simulink model "modeloNaoLinear"  (R2022a)
settings: Solver=FixedStepAuto  StartTime=0.0  StopTime=15  FixedStep=0.01  RelTol=1e-3
values from neighbouring files (symbols this model uses):
  CA = 8.564    [Identificacao.m]    (also in Linearizacao_CSTR.m)
  CAf = 10    [Identificacao.m]    (also in Linearizacao_CSTR.m)
  dCAf = 0    [Identificacao.m]    (also in Linearizacao_CSTR.m)
  dF = 0.01    [Identificacao.m]    (also in Linearizacao_CSTR.m)
  dTf = 0    [Identificacao.m]    (also in Linearizacao_CSTR.m)
  dTj = 0    [Identificacao.m]    (also in Linearizacao_CSTR.m)
  F = 1    [Identificacao.m]    (also in Linearizacao_CSTR.m)
  T = 311.2    [Identificacao.m]    (also in Linearizacao_CSTR.m; modeloDegrau.m = -Theta(3); parametrosFOPTD_igor.m = -Theta(3))
  Tf = 298    [Identificacao.m]    (also in Linearizacao_CSTR.m)
  Tj = 298    [Identificacao.m]    (also in Linearizacao_CSTR.m)
settings Model: Creator=veloc  LastModifiedBy=veloc

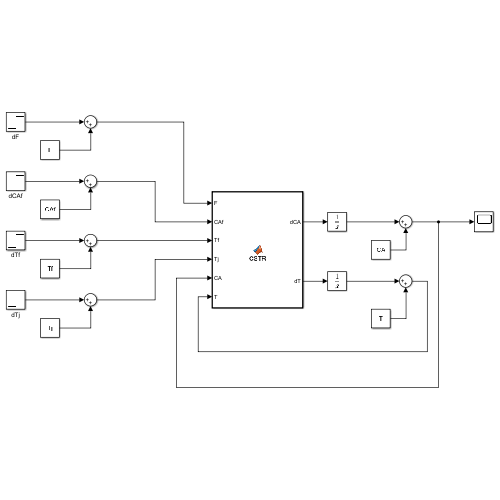
[thumbnail: Simulink's stored preview of the top-level diagram]
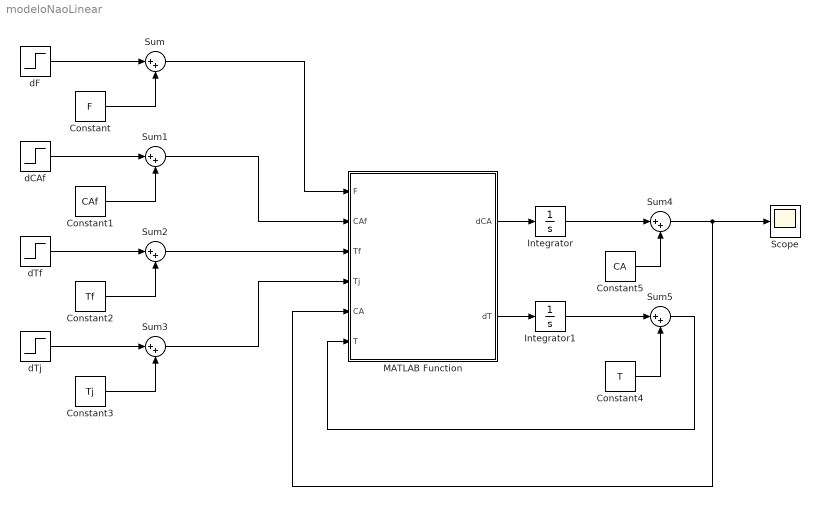
== system modeloNaoLinear ==
  Constant : Constant  Value=F
  Constant1 : Constant  Value=CAf
  Constant2 : Constant  Value=Tf
  Constant3 : Constant  Value=Tj
  Constant4 : Constant  Value=T
  Constant5 : Constant  Value=CA
  Integrator : Integrator
  Integrator1 : Integrator
  MATLAB Function : MATLAB Function  TreatAsAtomicUnit=on
  Scope : Scope
  Sum{,1..5} (6 alike) : Sum  Inputs=|++
  dCAf : Step  Time=0  Before=dCAf  SampleTime=0
  dF : Step  Time=0  After=dF  SampleTime=0
  dTf : Step  Time=0  After=dTf  SampleTime=0
  dTj : Step  Time=0  After=dTj  SampleTime=0
  wires:
  Sum3/1 -> MATLAB Function/4(Tj)
  Sum2/1 -> MATLAB Function/3(Tf)
  Sum1/1 -> MATLAB Function/2(CAf)
  Sum/1 -> MATLAB Function/1(F)
  Constant1/1 -> Sum1/2
  Constant/1 -> Sum/2
  Constant2/1 -> Sum2/2
  Constant3/1 -> Sum3/2
  Sum5/1 -> MATLAB Function/6(T)
  Constant4/1 -> Sum5/2
  Constant5/1 -> Sum4/2
  dF/1 -> Sum/1
  dCAf/1 -> Sum1/1
  dTf/1 -> Sum2/1
  dTj/1 -> Sum3/1
  Sum4/1 -> Scope/1, MATLAB Function/5(CA)
  MATLAB Function/2(dT) -> Integrator1/1
  MATLAB Function/1(dCA) -> Integrator/1
  Integrator/1 -> Sum4/1
  Integrator1/1 -> Sum5/1

== matlab function modeloNaoLinear/MATLAB Function ==
  data: F input; dCA output; CAf input; Tf input; Tj input; CA input; T input; dT output
function [dCA,dT] = CSTR(F, CAf, Tf, Tj, CA, T)
    % F: Vazão volumétrica
    % Caf: Concentração de A na alimentação
    % Tf: Temperatura da alimentação
    % Tj: Temperatura da jaqueta
    % V: Volume do reator
    % k0: Fator pré-exponencial
    % deltaE: Energia de ativação
    % R: Constante dos gases ideais
    % deltaH: Calor de reação
    % rho: Densidade
    % cp: Capacidade térmica
    % U: Coeficiente global de transferência de calor
    % A: Área de troca térmica

    % Parâmetros da simulação
    V = 1;  % m^3
    deltaE = 11843;  % J/mol
    pCp = 500;  % J/Km^3
    R = 1.987;  % L/molK
    UA = 150;  % J/Kh
    k0 = 9703 * 3600;  % h^-1
    deltaH = -5960;  % J/mol

    % Equação da taxa de reação (Arrhenius)
    r = k0*exp(-deltaE/(R*T))*CA;

%     % Equação diferencial para dCA/dt
%     dCAdt = (F / V) * (Caf - Ca) - r;
% 
%     % Equação diferencial para dT/dt
%     dTdt = (F / V) * (Tf-T) + (-deltaH/(rho_cp)*r)  - (UA/(V * rho_cp)) * (T - Tj);

    dCA = F/V*(CAf-CA)-r;
    dT = F/V*(Tf-T)+(-deltaH/(pCp)*r)-UA/(V*pCp)*(T-Tj);
